simulink model "mras_normalized_square_error"  (R2019b)
settings: Solver=VariableStepAuto  StartTime=0.0  StopTime=100  RelTol=1e-3
values from neighbouring files (symbols this model uses):
  alpha = 10    [Second_order_system.m]
  Am = [1 7 12]    [Second_order_system.m]
  b = 7    [Second_order_system.m]
  Bm = 12    [Second_order_system.m]
  gamma = 1.2    [Second_order_system.m]
settings Model: Creator=Mustafa Sezer  LastModifiedBy=Mustafa Sezer

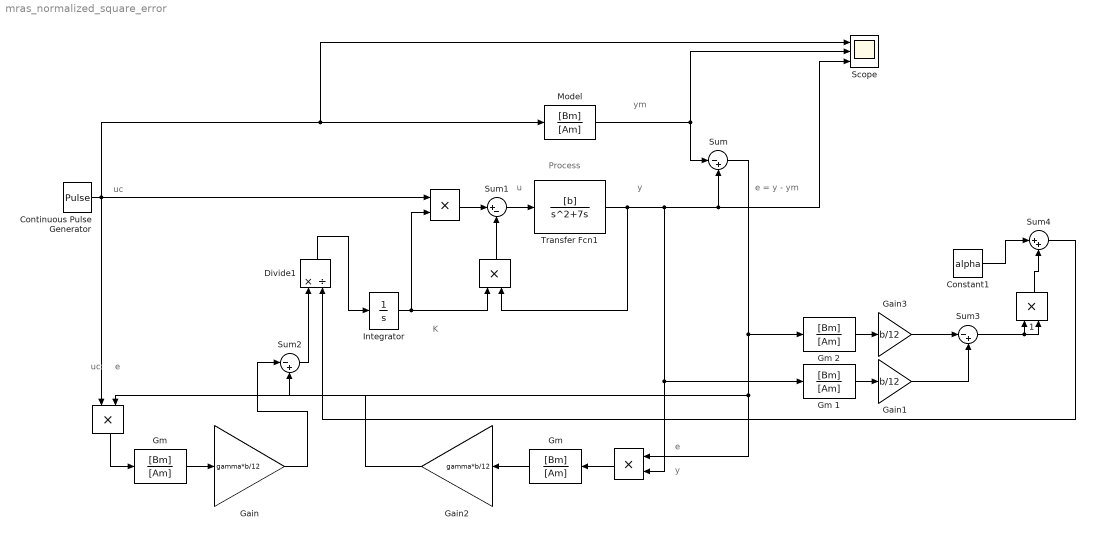
== system mras_normalized_square_error ==
  note: ym
  note: e = y - ym
  note: e
  note: u
  note: K
  note: uc
  note: Process
  note: y
  note: e
  note: uc
  note: y
   {,,,1} (4 alike) : Product
  "     " : Product
  Constant1 : Constant  Value=alpha
  Continuous Pulse Generator : DiscretePulseGenerator  PulseType=Time based  Amplitude=10  Period=20  PulseWidth=50
  Divide1 : Product  Inputs=*/
  Gain : Gain  Gain=gamma*b/12
  Gain1 : Gain  Gain=b/12
  Gain2 : Gain  Gain=gamma*b/12
  Gain3 : Gain  Gain=b/12
  "Gm " : TransferFcn  Numerator=[Bm]  Denominator=[Am]
  "Gm  " : TransferFcn  Numerator=[Bm]  Denominator=[Am]
  Gm 1 : TransferFcn  Numerator=[Bm]  Denominator=[Am]
  Gm 2 : TransferFcn  Numerator=[Bm]  Denominator=[Am]
  Integrator : Integrator
  Model : TransferFcn  Numerator=[Bm]  Denominator=[Am]
  Scope : Scope  NumInputPorts=3
  Sum : Sum  Inputs=|-+
  Sum1 : Sum  Inputs=|+-
  Sum2 : Sum  Inputs=|-+
  Sum3 : Sum  Inputs=|-+
  Sum4 : Sum  Inputs=|++
  Transfer Fcn1 : TransferFcn  Numerator=[b]  Denominator=[1 7 0]
  wires:
  " "/1 -> "Gm "/1
  Gain2/1 -> Sum2/2
  "Gm "/1 -> Gain2/1
  Gain/1 -> Sum2/1
  " "/1 -> Sum1/2
  Continuous Pulse Generator/1 -> "     "/1, Scope/1, Model/1, " "/1
  Integrator/1 -> " "/1, "     "/2
  Sum/1 -> Gm 2/1, " "/1, " "/2
  Sum1/1 -> Transfer Fcn1/1
  Model/1 -> Sum/1, Scope/2
  Transfer Fcn1/1 -> " "/2, Gm 1/1, Sum/2, Scope/3, " "/2
  "Gm  "/1 -> Gain/1
  "     "/1 -> Sum1/1
  " "/1 -> "Gm  "/1
  Sum2/1 -> Divide1/1
  Gm 1/1 -> Gain1/1
  Gain1/1 -> Sum3/2
  Gm 2/1 -> Gain3/1
  Gain3/1 -> Sum3/1
  Sum3/1 -> " 1"/2, " 1"/1
  Constant1/1 -> Sum4/1
  " 1"/1 -> Sum4/2
  Sum4/1 -> Divide1/2
  Divide1/1 -> Integrator/1
